simulink model "Lab5_Ex1"  (R2015a)
settings: Solver=ode45  StartTime=0.0  StopTime=500  FixedStep=0.0001  RelTol=1e-3
values from neighbouring files (symbols this model uses):
  C = 10*C/100    [RLC.m]    (also in RLC_COMPLEX.m = 10)
  L1 = 1    [RLC_COMPLEX.m]
  L2 = 2    [RLC_COMPLEX.m]
  R1 = 10    [RLC_COMPLEX.m]
  R2 = 20    [RLC_COMPLEX.m]
settings Model: Creator=Bilal  LastModifiedBy=Bilal

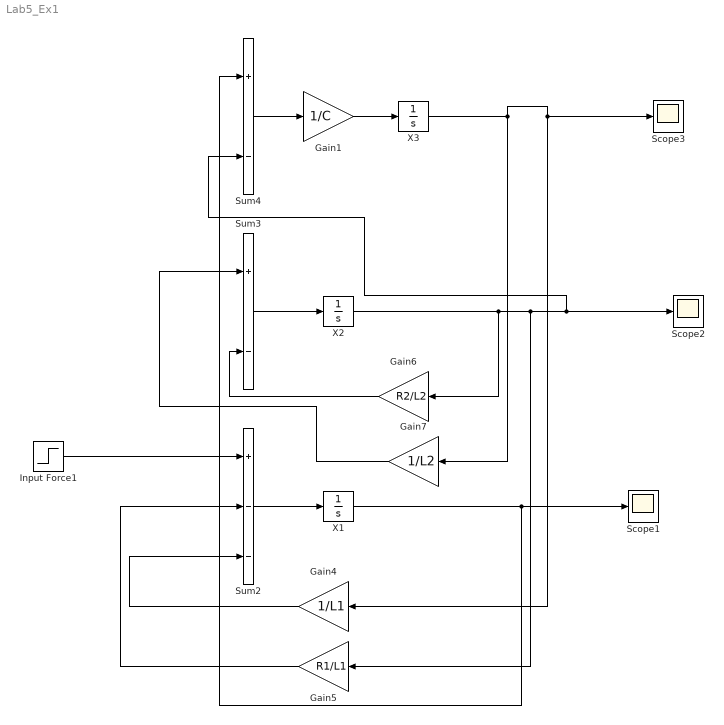
== system Lab5_Ex1 ==
  Gain1 : Gain  Gain=1/C
  Gain4 : Gain  Gain=1/L1
  Gain5 : Gain  Gain=R1/L1
  Gain6 : Gain  Gain=R2/L2
  Gain7 : Gain  Gain=1/L2
  Input Force1 : Step  After=E/L1
  Scope1 : Scope
      settings: ShowLegends=on  TimeRange=200  YMin=-200  YMax=200  MaxDataPoints=50000
  Scope2 : Scope
      settings: TimeRange=10  YMin=0  YMax=4  SaveName=ScopeData2
  Scope3 : Scope
      settings: YMin=0  YMax=80  SaveName=ScopeData3
  Sum2 : Sum  Inputs=+--
  Sum3 : Sum  Inputs=+-
  Sum4 : Sum  Inputs=+-
  X1 : Integrator
  X2 : Integrator
  "X3 " : Integrator
  wires:
  Sum2/1 -> X1/1
  Sum3/1 -> X2/1
  Sum4/1 -> Gain1/1
  Gain5/1 -> Sum2/2
  Gain4/1 -> Sum2/3
  Input Force1/1 -> Sum2/1
  Gain6/1 -> Sum3/2
  Gain7/1 -> Sum3/1
  X1/1 -> Sum4/1, Scope1/1
  X2/1 -> Sum4/2, Scope2/1, Gain5/1, Gain6/1
  "X3 "/1 -> Gain7/1, Scope3/1, Gain4/1
  Gain1/1 -> "X3 "/1
